simulink model "doublemass"  (R2022a)
settings: Solver=FixedStepAuto  StartTime=0.0  StopTime=20  FixedStep=0.0001  RelTol=1e-3
undefined symbols (not defined in the file): c1, c2, c3, k1, k2, k3, m1, m2
settings Model: Creator=mikol  LastModifiedBy=mikol

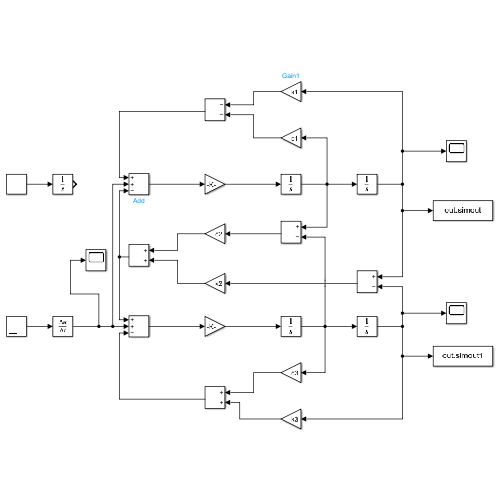
[thumbnail: Simulink's stored preview of the top-level diagram]
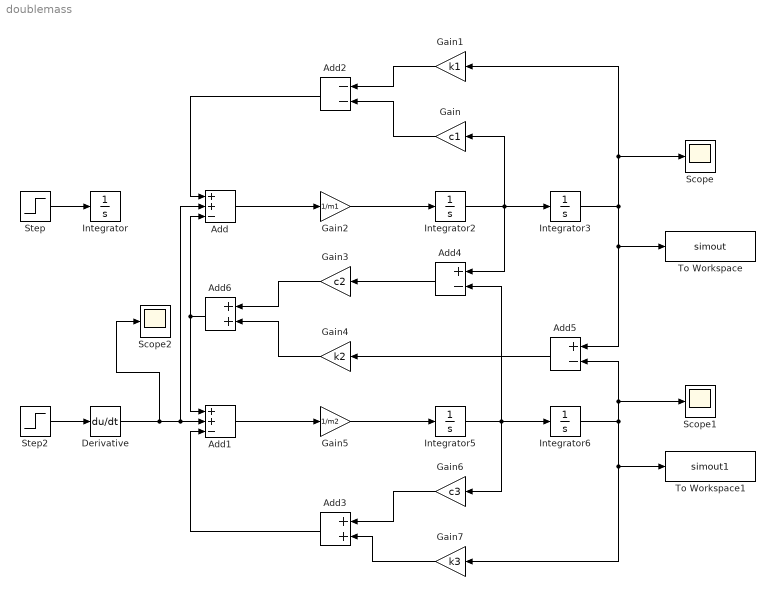
== system doublemass ==
  Add : Sum  Inputs=++-
  Add1 : Sum  Inputs=++-
  Add2 : Sum  Inputs=--
  Add3 : Sum
  Add4 : Sum  Inputs=+-
  Add5 : Sum  Inputs=+-
  Add6 : Sum
  Derivative : Derivative
  Gain : Gain  Gain=c1
  Gain1 : Gain  Gain=k1
  Gain2 : Gain  Gain=1/m1
  Gain3 : Gain  Gain=c2
  Gain4 : Gain  Gain=k2
  Gain5 : Gain  Gain=1/m2
  Gain6 : Gain  Gain=c3
  Gain7 : Gain  Gain=k3
  Integrator{,2..3,5..6} (5 alike) : Integrator
  Scope : Scope
  Scope1 : Scope
  Scope2 : Scope
  Step : Step  Time=0  SampleTime=0
  Step2 : Step  Time=0.0001  SampleTime=0
  To Workspace : ToWorkspace  VariableName=simout  SaveFormat=Timeseries  SampleTime=-1
  To Workspace1 : ToWorkspace  VariableName=simout1  SaveFormat=Timeseries  SampleTime=-1
  wires:
  Step/1 -> Integrator/1
  Add/1 -> Gain2/1
  Gain2/1 -> Integrator2/1
  Integrator2/1 -> Add4/1, Integrator3/1, Gain/1
  Integrator3/1 -> Add5/1, To Workspace/1, Scope/1, Gain1/1
  Add1/1 -> Gain5/1
  Gain5/1 -> Integrator5/1
  Integrator5/1 -> Gain6/1, Integrator6/1, Add4/2
  Integrator6/1 -> Gain7/1, To Workspace1/1, Add5/2, Scope1/1
  Gain1/1 -> Add2/1
  Gain/1 -> Add2/2
  Gain6/1 -> Add3/1
  Gain7/1 -> Add3/2
  Add2/1 -> Add/1
  Add5/1 -> Gain4/1
  Add4/1 -> Gain3/1
  Gain3/1 -> Add6/1
  Gain4/1 -> Add6/2
  Add6/1 -> Add1/1, Add/3
  Add3/1 -> Add1/3
  Step2/1 -> Derivative/1
  Derivative/1 -> Add1/2, Add/2, Scope2/1
